simulink model "im_test"  (R2024b)
settings: Solver=VariableStepAuto  StartTime=0.0  StopTime=10.0  RelTol=1e-3
libraries: peripheral_utilities x2, spsAsynchronousMachineSIUnitsLib x1, spsControlledVoltageSourceLib x1, gmp_sil_core_pack x1, spsGroundLib x1, sps_lib x1
settings Model: Creator=javnson  LastModifiedBy=javnson
settings OptimizationCC: ReuseModelBlockBuffer=off
settings RTWCC: GPUComputeCapability=3.5

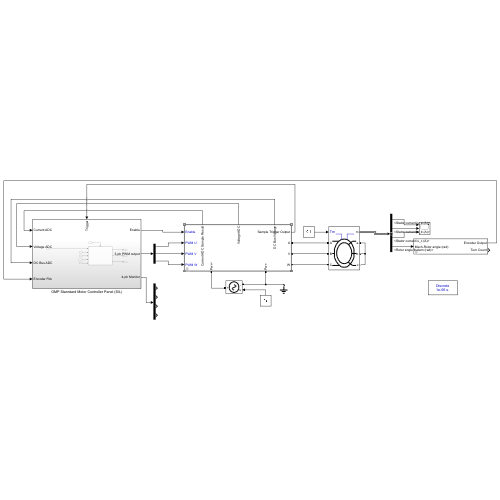
[thumbnail: Simulink's stored preview of the top-level diagram]
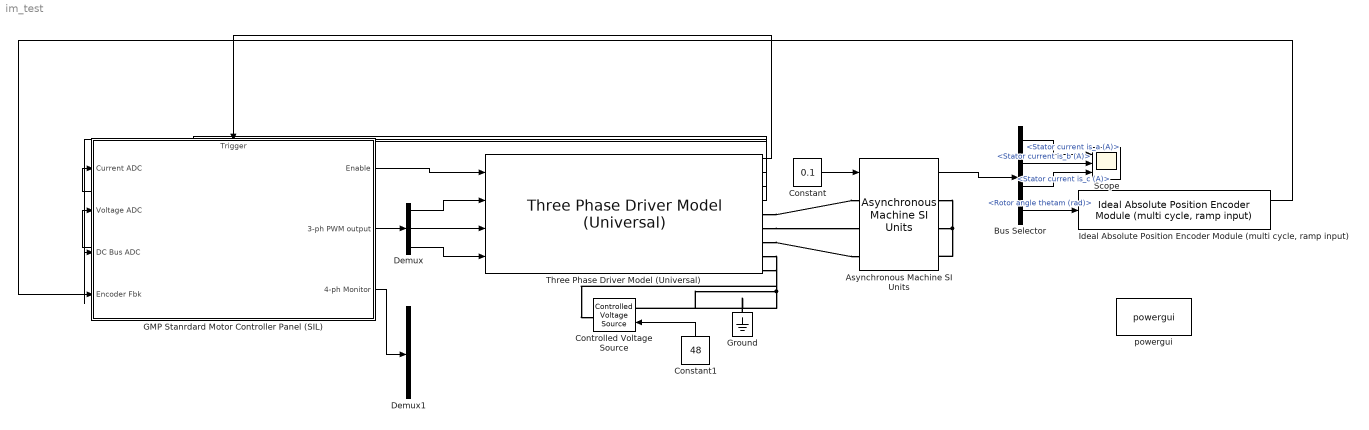
== system im_test ==
  Asynchronous Machine SI Units : spsAsynchronousMachineSIUnitsLib/Asynchronous Machine SI Units  RotorType=Wound  PresetModel=No  MechanicalLoad=Torque Tm  ShowDetailedParameters=on  ReferenceFrame=Rotor  Units=SI  MeasurementBus=off  NominalParameters=[1.845e+04 400 50]  VoltageRatio=1  Stator=[0.5968 0.0003495]  Rotor=[0.6258 0.005473]  Cage1=[0.4155 0.002066]  Cage2=[0.4168 0.0003495]  Lm=0.0354  Mechanical=[0.05 0.005879 2]  PolePairs=2  InitialConditions=[0 0 0 0 0 0 0 0]  SimulateSaturation=off  Saturation=[14.03593122, 27.81365428, 53.79336849, 72.68890987, 97.98006896, 148.6815601, 215.7428561, 302.9841135, 428.7778367 ; 230, 322, 414, 460, 506, 552, 598, 644, 690]  LoadFlowParameters=1492000  TsPowergui=0  TsBlock=-1  IterativeModel=Trapezoidal non iterative  IterativeDiscreteModel=Trapezoidal non iterative  Pmec=1.492e+006
  Bus Selector : BusSelector  OutputSignals=Stator measurements.Stator current is_a (A),Stator measurements.Stator current is_b (A),Stator measurements.Stator current is_c (A),Mechanical.Rotor angle thetam (rad)
  Constant : Constant  Value=0.1
  Constant1 : Constant  Value=48
  Controlled Voltage Source : spsControlledVoltageSourceLib/Controlled Voltage Source  Initialize=on  Source_Type=AC  Amplitude=0  Phase=0  Frequency=0  Measurements=None
  Demux : Demux  Outputs=3
  Demux1 : Demux
  GMP Stanrdard Motor Controller Panel (SIL) : Subsystem
      settings: PortSchema="{\"entries\":[{\"content\":{\"sides\":[{\"content\":{\"connectorIds\":[\"In1\",\"In2\",\"In3\",\"In4\"]},\"type\":\"ConnectorPlacement.EquallySpacedRectSide\",\"uuid\":\"92070e77-c4d8-4bd6-a20f-015d90d53703\"},{\"content\":{\"connectorIds\":[\"Out1\",\"Out2\",\"Out3\"],\"side\":\"RIGHT\"},\"type\":\"ConnectorPlacement.EquallySpacedRectSide\",\"uuid\":\"cd227558-01ea-4976-b12d-cc815f5c8239\"},{\"content\":{\"connectorIds\":[\"In5\"],\"side\":\"TOP\"},\"type\":\"ConnectorPlacement.EquallySpacedRectSide\",\"uuid\":\"6d86fdab-8964-4d81-bb99-d1a603f01c68\"}]},\"type\":\"ConnectorPlacement.EquallySpacedConnector\",\"uuid\":\"4dd76185-b108-46e1-8d6d-0c6e9edd0ad4\"}],\"packageUris\":[\"http://schema.mathworks.com/mf0/Connector/R2020b\"],\"version\":\"1.0\"}"
  Ground : spsGroundLib/Ground  LConnTagsString=a
  "Ideal Absolute Position Encoder Module (multi cycle, ramp input)" : peripheral_utilities/Ideal Absolute Position Encoder Module (multi cycle, ramp input)  ENCODER_BIT=17
      settings: SourceProductName=Virtual Peripheral Utilities
  Scope : Scope  NumInputPorts=3
  Three Phase Driver Model (Universal) : peripheral_utilities/Three Phase Driver Model (Universal)  fswitch=10e3  CMP_MAX=10000  Deadband_Upper=100  Deadband_Lower=100  Deadband_us=1  phase_shift=0  R_mosfet_on=0.1  Lon=0  Rd=0.01  Vf=0.3  Rs=1e5  Cs=inf  Rsap=0.1  ADC_GAIN=0.1  ADC_BIT=16  ADC_REFERENCE=3.0  ADC_BIAS=1.5  ADC_INIT=0  VOLTAGE_ADC_GAIN=1  VOLTAGE_ADC_BIT=16  VOLTAGE_ADC_REFERENCE=48  VOLTAGE_ADC_VOLTAGE=10  VOLTAGE_ADC_INIT=0  VOLTAGE_ADC_CUT_FREQ=500  DCBUS_ADC_GAIN=1  DCBUS_ADC_BIT=16  DCBUS_ADC_REFERENCE=48  DCBUS_ADC_BIAS=0  DCBUS_ADC_INIT=0
      settings: SourceProductName=Virtual Peripheral Utilities
  powergui : sps_lib/powergui  Priority=1  SimulationMode=Discrete  SampleTime=1e-6  frequency=60  Iterations=50  frequencyindice=50  Pbase=100e6  ErrMax=1e-4  UnitsV=kV  UnitsW=MW  buscounter=0  FunctionMessages=off  echomessages=off  EnableUseOfTLC=off  CurrentSourceSwitches=off  DisableSnubberDevices=off  DisableRonSwitches=off  DisableVfSwitches=off  DisplayEquations=off  AutomaticDiscreteSolvers=off  SolverType=Tustin/Backward Euler (TBE)  Interpol=off  ExternalGateDelay=off  methode=off  Ts=100  x0status=blocks  SPID=on  SwTol=0  HookPort=off  NonlinearTolerance=1e-4  nMaxIteration=100  ContinueOnMaxIteration=off  RestoreLinks=warning  ResistiveCurrentMeasurement=off  Frange=[0:2:500]  Ylog=off  Xlog=on  ShowGrid=off  save=off  variable=ZData  structure=0  ZoomFFT=off  StartTime=0.0  cycles=1  DisplayStyle=1  fundamental=60  FreqAxis=off  MaxFrequency=1000  frequencyindicesteady=1  RmsSteady=1  display=off
  wires:
  Constant/1 -> Asynchronous Machine SI Units/1
  Asynchronous Machine SI Units/1 -> Bus Selector/1
  Bus Selector/1 -> Scope/1  "<Stator current is_a (A)>"
  Bus Selector/2 -> Scope/2  "<Stator current is_b (A)>"
  Bus Selector/3 -> Scope/3  "<Stator current is_c (A)>"
  Demux/1 -> Three Phase Driver Model (Universal)/2
  Demux/2 -> Three Phase Driver Model (Universal)/3
  Demux/3 -> Three Phase Driver Model (Universal)/4
  Constant1/1 -> Controlled Voltage Source/1
  Bus Selector/4 -> "Ideal Absolute Position Encoder Module (multi cycle, ramp input)"/1  "<Rotor angle thetam (rad)>"
  Three Phase Driver Model (Universal)/2 -> GMP Stanrdard Motor Controller Panel (SIL)/1(Current ADC)
  Three Phase Driver Model (Universal)/3 -> GMP Stanrdard Motor Controller Panel (SIL)/2(Voltage ADC)
  "Ideal Absolute Position Encoder Module (multi cycle, ramp input)"/1 -> GMP Stanrdard Motor Controller Panel (SIL)/4(Encoder Fbk)
  GMP Stanrdard Motor Controller Panel (SIL)/1(Enable) -> Three Phase Driver Model (Universal)/1
  GMP Stanrdard Motor Controller Panel (SIL)/2(3-ph PWM output) -> Demux/1
  GMP Stanrdard Motor Controller Panel (SIL)/3(4-ph Monitor) -> Demux1/1
  Three Phase Driver Model (Universal)/1 -> GMP Stanrdard Motor Controller Panel (SIL)/5(Trigger)
  Three Phase Driver Model (Universal)/4 -> GMP Stanrdard Motor Controller Panel (SIL)/3(DC Bus ADC)
  connections:
  Three Phase Driver Model (Universal)/RConn1 -- Asynchronous Machine SI Units/LConn1
  Three Phase Driver Model (Universal)/RConn2 -- Asynchronous Machine SI Units/LConn2
  Three Phase Driver Model (Universal)/RConn3 -- Asynchronous Machine SI Units/LConn3
  Asynchronous Machine SI Units/RConn1 -- Asynchronous Machine SI Units/RConn2 -- Asynchronous Machine SI Units/RConn3
  Three Phase Driver Model (Universal)/RConn4 -- Controlled Voltage Source/RConn1
  Three Phase Driver Model (Universal)/RConn5 -- Controlled Voltage Source/LConn1 -- Ground/LConn1

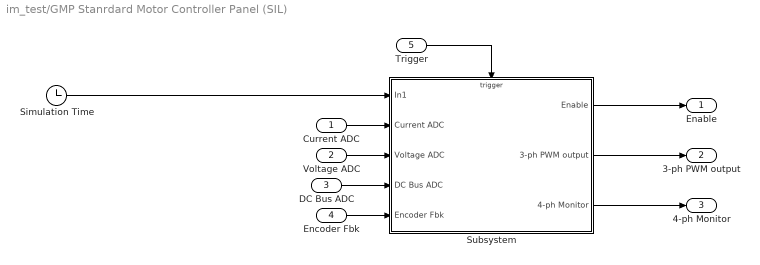
== system im_test/GMP Stanrdard Motor Controller Panel (SIL) ==
  Current ADC : Inport
  Voltage ADC : Inport  Port=2
  DC Bus ADC : Inport  Port=3
  Encoder Fbk : Inport  Port=4
  Trigger : Inport  Port=5
  Simulation Time : Clock
  Subsystem : Subsystem
  Enable : Outport
  3-ph PWM output : Outport  Port=2
  4-ph Monitor : Outport  Port=3
  wires:
  Simulation Time/1 -> Subsystem/1(In1)
  Current ADC/1 -> Subsystem/2(Current ADC)
  Voltage ADC/1 -> Subsystem/3(Voltage ADC)
  DC Bus ADC/1 -> Subsystem/4(DC Bus ADC)
  Encoder Fbk/1 -> Subsystem/5(Encoder Fbk)
  Subsystem/1(Enable) -> Enable/1
  Subsystem/2(3-ph PWM output) -> 3-ph PWM output/1
  Subsystem/3(4-ph Monitor) -> 4-ph Monitor/1
  Trigger/1 -> Subsystem/Trigger

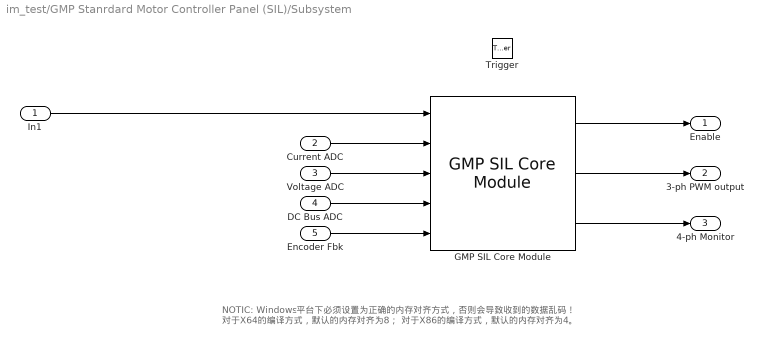
== system im_test/GMP Stanrdard Motor Controller Panel (SIL)/Subsystem ==
  note: NOTIC:
      | Windows平台下必须设置为正确的内存对齐方式，否则会导致收到的数据乱码！
      | 对于X64的编译方式，默认的内存对齐为8；
      | 对于X86的编译方式，默认的内存对齐为4。
  In1 : Inport
  Current ADC : Inport  Port=2
  Voltage ADC : Inport  Port=3
  DC Bus ADC : Inport  Port=4
  Encoder Fbk : Inport  Port=5
  Trigger : TriggerPort  VariantControl=(inherit)  PortDimensions=1
  GMP SIL Core Module : gmp_sil_core_pack/GMP SIL Core Module  MaskPackedDataTypes={'double','uint32','uint32','uint32','uint32'}  MaskPackedDataSizes={[1],[3],[3],[1],[1]}  MaskUnpackedDataTypes={'double', 'uint32','double'}  MaskUnpackedDataSizes={[1],[3],[4]}  MaskAlignment=1  MaskHostAddr='127.0.0.1'  MaskMsgTxPort=12300  MaskMsgRxPort=12301  MaskCmdTxPort=12302  MaskCmdRxPort=12303
      settings: SourceProductName=GMP SIL Core Utilities
  Enable : Outport
  3-ph PWM output : Outport  Port=2
  4-ph Monitor : Outport  Port=3
  wires:
  Encoder Fbk/1 -> GMP SIL Core Module/5
  Current ADC/1 -> GMP SIL Core Module/2
  Voltage ADC/1 -> GMP SIL Core Module/3
  DC Bus ADC/1 -> GMP SIL Core Module/4
  In1/1 -> GMP SIL Core Module/1
  GMP SIL Core Module/3 -> 4-ph Monitor/1
  GMP SIL Core Module/2 -> 3-ph PWM output/1
  GMP SIL Core Module/1 -> Enable/1
